simulink model "INELFE"  (R2023b)
settings: Solver=ode1  StartTime=0.0  StopTime=sim_config.Tsim  RelTol=1e-3
undefined symbols (not defined in the file): sim_config
libraries: myLibrary x19, spsThreePhaseVIMeasurementLib x9, spsPower3phInstantaneousLib x5, spspowerguiLib x1
settings Model: Creator=dionm  LastModifiedBy=dionm

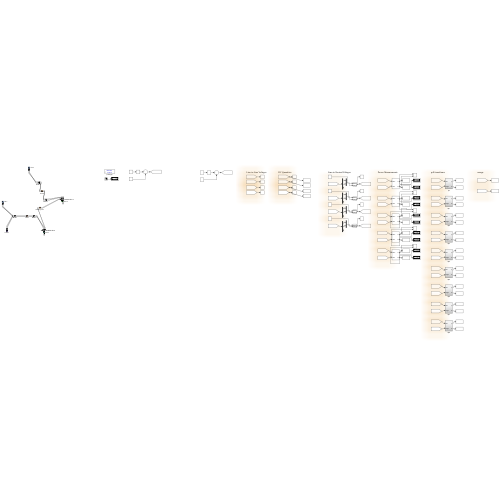
[thumbnail: Simulink's stored preview of the top-level diagram]
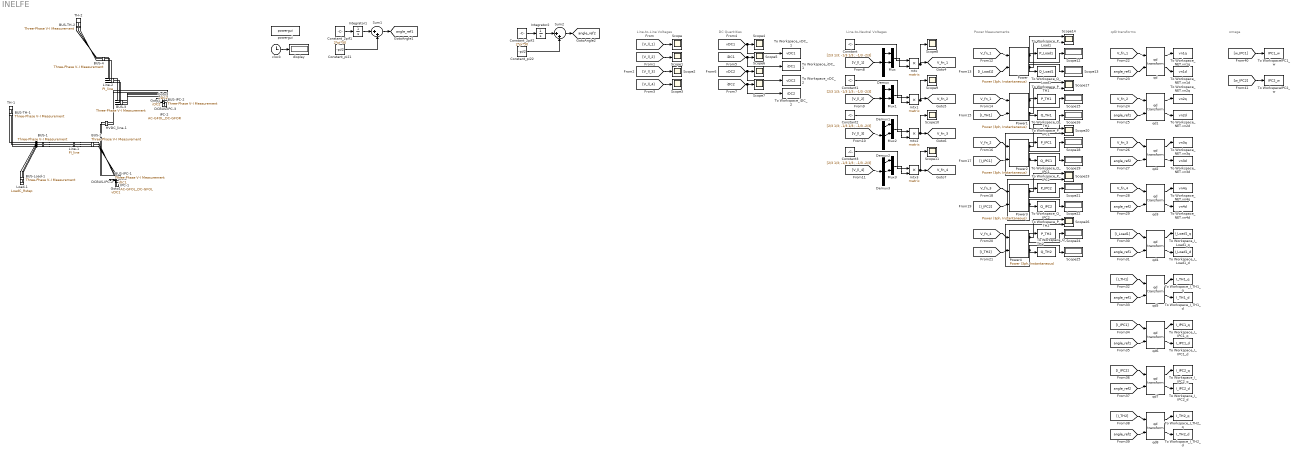
== system INELFE ==
  note: Line-to-Line Voltages
  note: DC Quantities
  note: Line-to-Neutral Voltages
  note: Power Measurements
  note: qd0 transforms
  note: omega
  BUS-1 : spsThreePhaseVIMeasurementLib/Three-Phase V-I Measurement  VoltageMeasurement=phase-to-phase  SetLabelV=on  LabelV=V_ll_1  Vpu=off  VpuLL=off  CurrentMeasurement=yes  SetLabelI=on  LabelI=I_1  Ipu=off  Pbase=100e6  Vbase=500e3  OutputType=Complex  PhasorSimulation=off  PSBequivalent=0
  BUS-2 : spsThreePhaseVIMeasurementLib/Three-Phase V-I Measurement  VoltageMeasurement=phase-to-phase  SetLabelV=on  LabelV=V_ll_2  Vpu=off  VpuLL=off  CurrentMeasurement=yes  SetLabelI=on  LabelI=I_2  Ipu=off  Pbase=100e6  Vbase=500e3  OutputType=Complex  PhasorSimulation=off  PSBequivalent=0
  BUS-3 : spsThreePhaseVIMeasurementLib/Three-Phase V-I Measurement  VoltageMeasurement=phase-to-phase  SetLabelV=on  LabelV=V_ll_3  Vpu=off  VpuLL=off  CurrentMeasurement=yes  SetLabelI=on  LabelI=I_3  Ipu=off  Pbase=100e6  Vbase=500e3  OutputType=Complex  PhasorSimulation=off  PSBequivalent=0
  BUS-4 : spsThreePhaseVIMeasurementLib/Three-Phase V-I Measurement  VoltageMeasurement=phase-to-phase  SetLabelV=on  LabelV=V_ll_4  Vpu=off  VpuLL=off  CurrentMeasurement=yes  SetLabelI=on  LabelI=I_4  Ipu=off  Pbase=100e6  Vbase=500e3  OutputType=Complex  PhasorSimulation=off  PSBequivalent=0
  BUS-IPC-1 : spsThreePhaseVIMeasurementLib/Three-Phase V-I Measurement  VoltageMeasurement=phase-to-phase  SetLabelV=on  LabelV=V_IPC_1  Vpu=off  VpuLL=off  CurrentMeasurement=yes  SetLabelI=on  LabelI=I_IPC1  Ipu=off  Pbase=100e6  Vbase=500e3  OutputType=Complex  PhasorSimulation=off  PSBequivalent=0
  BUS-IPC-2 : spsThreePhaseVIMeasurementLib/Three-Phase V-I Measurement  VoltageMeasurement=phase-to-phase  SetLabelV=on  LabelV=V_IPC_2  Vpu=off  VpuLL=off  CurrentMeasurement=yes  SetLabelI=on  LabelI=I_IPC2  Ipu=off  Pbase=100e6  Vbase=500e3  OutputType=Complex  PhasorSimulation=off  PSBequivalent=0
  BUS-Load-1 : spsThreePhaseVIMeasurementLib/Three-Phase V-I Measurement  VoltageMeasurement=phase-to-phase  SetLabelV=on  LabelV=V_Load_1  Vpu=off  VpuLL=off  CurrentMeasurement=yes  SetLabelI=on  LabelI=I_Load1  Ipu=off  Pbase=100e6  Vbase=500e3  OutputType=Complex  PhasorSimulation=off  PSBequivalent=0
  BUS-TH-1 : spsThreePhaseVIMeasurementLib/Three-Phase V-I Measurement  VoltageMeasurement=phase-to-phase  SetLabelV=on  LabelV=V_TH_1  Vpu=off  VpuLL=off  CurrentMeasurement=yes  SetLabelI=on  LabelI=I_TH1  Ipu=off  Pbase=100e6  Vbase=500e3  OutputType=Complex  PhasorSimulation=off  PSBequivalent=0
  BUS-TH-2 : spsThreePhaseVIMeasurementLib/Three-Phase V-I Measurement  VoltageMeasurement=phase-to-phase  SetLabelV=on  LabelV=V_TH_2  Vpu=off  VpuLL=off  CurrentMeasurement=yes  SetLabelI=on  LabelI=I_TH2  Ipu=off  Pbase=100e6  Vbase=500e3  OutputType=Complex  PhasorSimulation=off  PSBequivalent=0
  Constant{,1..3} (4 alike) : Constant  Value=[2/3 1/3; -1/3 1/3 ; -1/3 -2/3]
  Constant_2pif1 : Constant  Value=2*pi*50
  Constant_2pif2 : Constant  Value=2*pi*50
  Constant_pi21 : Constant  Value=-pi/2
  Constant_pi22 : Constant  Value=-pi/2
  DCBUS-IPC-2 : myLibrary/DCBUS  SystemSampleTime=-1  VariantActivationTime=update diagram  AllowFlexibleInterface=on  Latency=0  AutoFrameSizeCalculation=off
  DCBUS-IPC-3 : myLibrary/DCBUS  SystemSampleTime=-1  VariantActivationTime=update diagram  AllowFlexibleInterface=on  Latency=0  AutoFrameSizeCalculation=off
  Demux{,1..3} (4 alike) : Demux  Outputs=3
  HVDC_line-1 : myLibrary/HVDC_line  T_HVDC_line_global=T_DC_NET  initDCLine_global=init_DCline  num=1
  IPC-1 : myLibrary/AC-GFOL_DC-GFOL  T_IPC_global=T_IPC  initIPC_global=init_IPC  num=1
  IPC-2 : myLibrary/AC-GFOL_DC-GFOR  T_IPC_global=T_IPC  initIPC_global=init_IPC  num=2
  Integrator1 : Integrator
  Integrator2 : Integrator
  Line-1 : myLibrary/PI_line  T_line_global=T_NET  initLine_global=init_line  num=1  set_C0=ones(1,6)  set_iL0=0
  Line-2 : myLibrary/PI_line  T_line_global=T_NET  initLine_global=init_line  num=2  set_C0=ones(1,6)  set_iL0=0
  Load-1 : myLibrary/LoadC_Rstep  T_load_global=T_load  initLoad_global=init_load  num=1  tstep=sim_config.tstep  Radd=Rload_add
  Mux{,1..3} (4 alike) : Mux  Inputs=2
  Power{,1..4} (5 alike) : spsPower3phInstantaneousLib/Power (3ph, Instantaneous)
  Scope{,1..11} (12 alike) : Scope
  Scope{12..13,15..16,18..19,21..22,24..25} (10 alike) : Display
  Scope{14,17,20,23,26} (5 alike) : Scope  NumInputPorts=2
  Sum1 : Sum  Inputs=|++
  Sum2 : Sum  Inputs=|++
  TH-1 : myLibrary/TH  T_TH_global=T_TH  initTH_global=init_TH  num=1
  TH-2 : myLibrary/TH  T_TH_global=T_TH  initTH_global=init_TH  num=2
  To WorkspaceIPC1_w : ToWorkspace  VariableName=IPC1_w  SampleTime=sim_config.Tsample
  To WorkspaceIPC2_w : ToWorkspace  VariableName=IPC2_w  SampleTime=sim_config.Tsample
  To Workspace_I_IPC1_d : ToWorkspace  VariableName=I_IPC1_d  SampleTime=sim_config.Tsample
  To Workspace_I_IPC1_q : ToWorkspace  VariableName=I_IPC1_q  SampleTime=sim_config.Tsample
  To Workspace_I_IPC2_d : ToWorkspace  VariableName=I_IPC2_d  SampleTime=sim_config.Tsample
  To Workspace_I_IPC2_q : ToWorkspace  VariableName=I_IPC2_q  SampleTime=sim_config.Tsample
  To Workspace_I_Load1_d : ToWorkspace  VariableName=I_Load1_d  SampleTime=sim_config.Tsample
  To Workspace_I_Load1_q : ToWorkspace  VariableName=I_Load1_q  SampleTime=sim_config.Tsample
  To Workspace_I_TH1_d : ToWorkspace  VariableName=I_TH1_d  SampleTime=sim_config.Tsample
  To Workspace_I_TH1_q : ToWorkspace  VariableName=I_TH1_q  SampleTime=sim_config.Tsample
  To Workspace_I_TH2_d : ToWorkspace  VariableName=I_TH2_d  SampleTime=sim_config.Tsample
  To Workspace_I_TH2_q : ToWorkspace  VariableName=I_TH2_q  SampleTime=sim_config.Tsample
  To Workspace_NET.vn1d : ToWorkspace  VariableName=vn1d  SampleTime=sim_config.Tsample
  To Workspace_NET.vn1q : ToWorkspace  VariableName=vn1q  SampleTime=sim_config.Tsample
  To Workspace_NET.vn2d : ToWorkspace  VariableName=vn2d  SampleTime=sim_config.Tsample
  To Workspace_NET.vn2q : ToWorkspace  VariableName=vn2q  SampleTime=sim_config.Tsample
  To Workspace_NET.vn3d : ToWorkspace  VariableName=vn3d  SampleTime=sim_config.Tsample
  To Workspace_NET.vn3q : ToWorkspace  VariableName=vn3q  SampleTime=sim_config.Tsample
  To Workspace_NET.vn4d : ToWorkspace  VariableName=vn4d  SampleTime=sim_config.Tsample
  To Workspace_NET.vn4q : ToWorkspace  VariableName=vn4q  SampleTime=sim_config.Tsample
  To Workspace_P_IPC1 : ToWorkspace  VariableName=P_IPC1  SampleTime=sim_config.Tsample
  To Workspace_P_IPC2 : ToWorkspace  VariableName=P_IPC2  SampleTime=sim_config.Tsample
  To Workspace_P_Load1 : ToWorkspace  VariableName=P_Load1  SampleTime=sim_config.Tsample
  To Workspace_P_TH1 : ToWorkspace  VariableName=P_TH1  SampleTime=sim_config.Tsample
  To Workspace_P_TH2 : ToWorkspace  VariableName=P_TH2  SampleTime=sim_config.Tsample
  To Workspace_Q_IPC1 : ToWorkspace  VariableName=Q_IPC1  SampleTime=sim_config.Tsample
  To Workspace_Q_IPC2 : ToWorkspace  VariableName=Q_IPC2  SampleTime=sim_config.Tsample
  To Workspace_Q_Load1 : ToWorkspace  VariableName=Q_Load1  SampleTime=sim_config.Tsample
  To Workspace_Q_TH1 : ToWorkspace  VariableName=Q_TH1  SampleTime=sim_config.Tsample
  To Workspace_Q_TH2 : ToWorkspace  VariableName=Q_TH2  SampleTime=sim_config.Tsample
  To Workspace_iDC_1 : ToWorkspace  VariableName=iDC1  SampleTime=sim_config.Tsample
  To Workspace_iDC_2 : ToWorkspace  VariableName=iDC2  SampleTime=sim_config.Tsample
  To Workspace_vDC_1 : ToWorkspace  VariableName=vDC1  SampleTime=sim_config.Tsample
  To Workspace_vDC_2 : ToWorkspace  VariableName=vDC2  SampleTime=sim_config.Tsample
  clock : Clock
  display : Display
  mtx{,1..3} (4 alike) : Product  Multiplication=Matrix(*)
  powergui : spspowerguiLib/powergui  Priority=1  SimulationMode=Discrete  SampleTime=sim_config.Ts  frequency=60  Iterations=50  frequencyindice=50  Pbase=100e6  ErrMax=1e-4  UnitsV=kV  UnitsW=MW  buscounter=0  FunctionMessages=off  echomessages=off  EnableUseOfTLC=off  CurrentSourceSwitches=off  DisableSnubberDevices=off  DisableRonSwitches=off  DisableVfSwitches=off  DisplayEquations=off  AutomaticDiscreteSolvers=off  SolverType=Tustin/Backward Euler (TBE)  Interpol=off  ExternalGateDelay=off  methode=off  Ts=100  x0status=blocks  SPID=on  SwTol=0  HookPort=off  NonlinearTolerance=1e-4  nMaxIteration=100  ContinueOnMaxIteration=off  RestoreLinks=warning  ResistiveCurrentMeasurement=off  Frange=[0:2:500]  Ylog=off  Xlog=on  ShowGrid=off  save=off  variable=ZData  structure=0  ZoomFFT=off  StartTime=0.0  cycles=1  DisplayStyle=1  fundamental=60  FreqAxis=off  MaxFrequency=1000  frequencyindicesteady=1  RmsSteady=1  display=off
  qd{,1..8} (9 alike) : myLibrary/qd transform  SystemSampleTime=-1  VariantActivationTime=update diagram  AllowFlexibleInterface=on  Latency=0  AutoFrameSizeCalculation=off
  tag scope: V_fn_1=global, V_fn_2=global, V_fn_3=global, V_fn_4=global, angle_ref1=global, angle_ref2=global, iDC1=global, iDC2=global, vDC1=global, vDC2=global
  wires:
  DCBUS-IPC-2/1 -> [iDC1]
  DCBUS-IPC-2/2 -> [vDC1]
  DCBUS-IPC-3/1 -> [iDC2]
  DCBUS-IPC-3/2 -> [vDC2]
  clock/1 -> display/1
  Constant_2pif1/1 -> Integrator1/1
  Integrator1/1 -> Sum1/1
  Constant_pi21/1 -> Sum1/2
  Sum1/1 -> [angle_ref1]
  Constant_2pif2/1 -> Integrator2/1
  Integrator2/1 -> Sum2/1
  Constant_pi22/1 -> Sum2/2
  Sum2/1 -> [angle_ref2]
  [V_ll_1] -> Scope/1
  [V_ll_2] -> Scope1/1
  [V_ll_3] -> Scope2/1
  [V_ll_4] -> Scope3/1
  [vDC1] -> Scope4/1, To Workspace_vDC_1/1
  [iDC1] -> Scope5/1, To Workspace_iDC_1/1
  [vDC2] -> Scope6/1, To Workspace_vDC_2/1
  [iDC2] -> Scope7/1, To Workspace_iDC_2/1
  [V_ll_1] -> Demux/1
  Demux/1 -> Mux/1
  Demux/2 -> Mux/2
  Mux/1 -> mtx/2
  Constant/1 -> mtx/1
  mtx/1 -> [V_fn_1], Scope8/1
  [V_ll_2] -> Demux1/1
  Demux1/1 -> Mux1/1
  Demux1/2 -> Mux1/2
  Mux1/1 -> mtx1/2
  Constant1/1 -> mtx1/1
  mtx1/1 -> [V_fn_2], Scope9/1
  [V_ll_3] -> Demux2/1
  Demux2/1 -> Mux2/1
  Demux2/2 -> Mux2/2
  Mux2/1 -> mtx2/2
  Constant2/1 -> mtx2/1
  mtx2/1 -> [V_fn_3], Scope10/1
  [V_ll_4] -> Demux3/1
  Demux3/1 -> Mux3/1
  Demux3/2 -> Mux3/2
  Mux3/1 -> mtx3/2
  Constant3/1 -> mtx3/1
  mtx3/1 -> [V_fn_4], Scope11/1
  [V_fn_1] -> Power/1
  [I_Load1] -> Power/2
  Power/1 -> To Workspace_P_Load1/1, Scope12/1, Scope14/1
  Power/2 -> To Workspace_Q_Load1/1, Scope13/1, Scope14/2
  [V_fn_1] -> Power1/1
  [I_TH1] -> Power1/2
  Power1/1 -> To Workspace_P_TH1/1, Scope15/1, Scope17/1
  Power1/2 -> To Workspace_Q_TH1/1, Scope16/1, Scope17/2
  [V_fn_2] -> Power2/1
  [I_IPC1] -> Power2/2
  Power2/1 -> To Workspace_P_IPC1/1, Scope18/1, Scope20/1
  Power2/2 -> To Workspace_Q_IPC1/1, Scope19/1, Scope20/2
  [V_fn_3] -> Power3/1
  [I_IPC2] -> Power3/2
  Power3/1 -> To Workspace_P_IPC2/1, Scope21/1, Scope23/1
  Power3/2 -> To Workspace_Q_IPC2/1, Scope22/1, Scope23/2
  [V_fn_4] -> Power4/1
  [I_TH2] -> Power4/2
  Power4/1 -> To Workspace_P_TH2/1, Scope24/1, Scope26/1
  Power4/2 -> To Workspace_Q_TH2/1, Scope25/1, Scope26/2
  [V_fn_1] -> qd/1
  [angle_ref1] -> qd/2
  qd/1 -> To Workspace_NET.vn1q/1
  qd/2 -> To Workspace_NET.vn1d/1
  [V_fn_2] -> qd1/1
  [angle_ref1] -> qd1/2
  qd1/1 -> To Workspace_NET.vn2q/1
  qd1/2 -> To Workspace_NET.vn2d/1
  [V_fn_3] -> qd2/1
  [angle_ref2] -> qd2/2
  qd2/1 -> To Workspace_NET.vn3q/1
  qd2/2 -> To Workspace_NET.vn3d/1
  [V_fn_4] -> qd3/1
  [angle_ref2] -> qd3/2
  qd3/1 -> To Workspace_NET.vn4q/1
  qd3/2 -> To Workspace_NET.vn4d/1
  [I_Load1] -> qd4/1
  [angle_ref1] -> qd4/2
  qd4/1 -> To Workspace_I_Load1_q/1
  qd4/2 -> To Workspace_I_Load1_d/1
  [I_TH1] -> qd5/1
  [angle_ref1] -> qd5/2
  qd5/1 -> To Workspace_I_TH1_q/1
  qd5/2 -> To Workspace_I_TH1_d/1
  [I_IPC1] -> qd6/1
  [angle_ref1] -> qd6/2
  qd6/1 -> To Workspace_I_IPC1_q/1
  qd6/2 -> To Workspace_I_IPC1_d/1
  [I_IPC2] -> qd7/1
  [angle_ref2] -> qd7/2
  qd7/1 -> To Workspace_I_IPC2_q/1
  qd7/2 -> To Workspace_I_IPC2_d/1
  [I_TH2] -> qd8/1
  [angle_ref2] -> qd8/2
  qd8/1 -> To Workspace_I_TH2_q/1
  qd8/2 -> To Workspace_I_TH2_d/1
  [w_IPC1] -> To WorkspaceIPC1_w/1
  [w_IPC2] -> To WorkspaceIPC2_w/1
  connections:
  BUS-2/RConn1 -- BUS-IPC-1/RConn1
  BUS-2/RConn2 -- BUS-IPC-1/RConn2
  BUS-2/RConn3 -- BUS-IPC-1/RConn3
  BUS-IPC-1/LConn1 -- IPC-1/RConn1
  BUS-IPC-1/LConn2 -- IPC-1/RConn2
  BUS-IPC-1/LConn3 -- IPC-1/RConn3
  DCBUS-IPC-2/LConn1 -- IPC-1/LConn1
  DCBUS-IPC-2/LConn2 -- IPC-1/LConn2
  BUS-3/RConn1 -- BUS-IPC-2/RConn1
  BUS-3/RConn2 -- BUS-IPC-2/RConn2
  BUS-3/RConn3 -- BUS-IPC-2/RConn3
  BUS-IPC-2/LConn1 -- IPC-2/RConn1
  BUS-IPC-2/LConn2 -- IPC-2/RConn2
  BUS-IPC-2/LConn3 -- IPC-2/RConn3
  DCBUS-IPC-3/LConn1 -- IPC-2/LConn1
  DCBUS-IPC-3/LConn2 -- IPC-2/LConn2
  DCBUS-IPC-2/RConn1 -- HVDC_line-1/LConn1
  DCBUS-IPC-2/RConn2 -- HVDC_line-1/LConn2
  HVDC_line-1/RConn1 -- DCBUS-IPC-3/RConn1
  HVDC_line-1/RConn2 -- DCBUS-IPC-3/RConn2
  BUS-4/LConn1 -- BUS-TH-2/RConn1
  BUS-4/LConn2 -- BUS-TH-2/RConn2
  BUS-4/LConn3 -- BUS-TH-2/RConn3
  BUS-TH-2/LConn1 -- TH-2/RConn1
  BUS-TH-2/LConn2 -- TH-2/RConn2
  BUS-TH-2/LConn3 -- TH-2/RConn3
  BUS-3/LConn1 -- Line-2/LConn1
  BUS-3/LConn2 -- Line-2/LConn2
  BUS-3/LConn3 -- Line-2/LConn3
  Line-2/RConn1 -- BUS-4/RConn1
  Line-2/RConn2 -- BUS-4/RConn2
  Line-2/RConn3 -- BUS-4/RConn3
  BUS-Load-1/LConn1 -- BUS-1/LConn1 -- BUS-TH-1/RConn1
  BUS-Load-1/LConn2 -- BUS-1/LConn2 -- BUS-TH-1/RConn2
  BUS-Load-1/LConn3 -- BUS-1/LConn3 -- BUS-TH-1/RConn3
  BUS-Load-1/RConn1 -- Load-1/LConn1
  BUS-Load-1/RConn2 -- Load-1/LConn2
  BUS-Load-1/RConn3 -- Load-1/LConn3
  BUS-TH-1/LConn1 -- TH-1/RConn1
  BUS-TH-1/LConn2 -- TH-1/RConn2
  BUS-TH-1/LConn3 -- TH-1/RConn3
  BUS-1/RConn1 -- Line-1/LConn1
  BUS-1/RConn2 -- Line-1/LConn2
  BUS-1/RConn3 -- Line-1/LConn3
  Line-1/RConn1 -- BUS-2/LConn1
  Line-1/RConn2 -- BUS-2/LConn2
  Line-1/RConn3 -- BUS-2/LConn3
